simulink model "dampers"  (R2021a)
settings: Solver=VariableStepAuto  StartTime=0.0  StopTime=10.0  RelTol=1e-3
undefined symbols (not defined in the file or in its folder): B_hs, gn, gp, K_hs, M, M_L
libraries: simulink x1
settings Model: Creator=artof  LastModifiedBy=artof

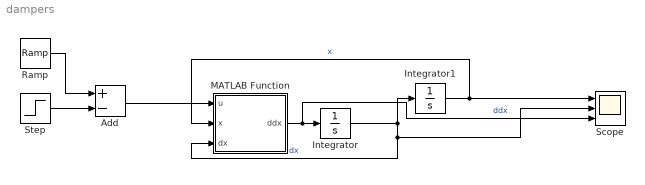
== system dampers ==
  Add : Sum  Inputs=+-
  Integrator : Integrator
  Integrator1 : Integrator
  MATLAB Function : MATLAB Function  TreatAsAtomicUnit=on
  Ramp : simulink/Sources/Ramp  slope=100  start=1  InitialOutput=0
  Scope : Scope  NumInputPorts=3
  Step : Step  Time=0  After=20  SampleTime=0
  wires:
  Integrator/1 -> Integrator1/1, MATLAB Function/3(dx), Scope/2  "dx"
  MATLAB Function/1(ddx) -> Scope/3, Integrator/1  "ddx"
  Integrator1/1 -> Scope/1, MATLAB Function/2(x)  "x"
  Ramp/1 -> Add/1
  Add/1 -> MATLAB Function/1(u)
  Step/1 -> Add/2

== matlab function dampers/MATLAB Function ==
  data: u input; ddx output; x input; dx input; K_hs parameter; B_hs parameter; gp parameter; gn parameter; M parameter; M_L parameter
function ddx = fcn(u, x, dx, K_hs, B_hs, gp, gn, M, M_L)

% Hard Stop
up_force = K_hs*(x-gp) + B_hs*dx*ge(dx,0);
bot_force = K_hs*(x-gn) + B_hs*dx*le(dx,0);
% up_force = K_hs*(x-gp) + B_hs*dx*abs(x-gp);
% bot_force = K_hs*(x-gn) + B_hs*dx*abs(x-gn);

% Dead zone calculating Hard Stop
if x >= gp
    F_hs = up_force;
elseif x > gn
    F_hs = 0;
else
    F_hs = bot_force;
end
F_g = (M + M_L)*9.81;
 

ddx = 1/(M+M_L)*(-F_hs - F_g + u);
